simulink model "mechanization_ell_earth_noise"  (R2025b)
settings: Solver=VariableStepAuto  StartTime=0.0  StopTime=time(end)  RelTol=1e-3
values from neighbouring files (symbols this model uses):
  pqr = omega_n    [test_traj_gen_v2 1.m]    (also in test_traj_gen_v2.m)
  rpy = zeros(length(time),3)    [test_traj_gen_v2 1.m]    (also in test_traj_gen_v2.m)
  ST = 1/100    (= 0.01)    [test_traj_gen_v2 1.m]    (also in test_traj_gen_v2.m)
  vel_n = vel_n_f    [test_traj_gen_v2 1.m]    (also in test_traj_gen_v2.m)
undefined symbols (not defined in the file or in its folder): DiscIntNeverNeededParam
settings Model: Creator=Lorenzo  LastModifiedBy=roly2
settings RTWCC: GPUComputeCapability=3.5

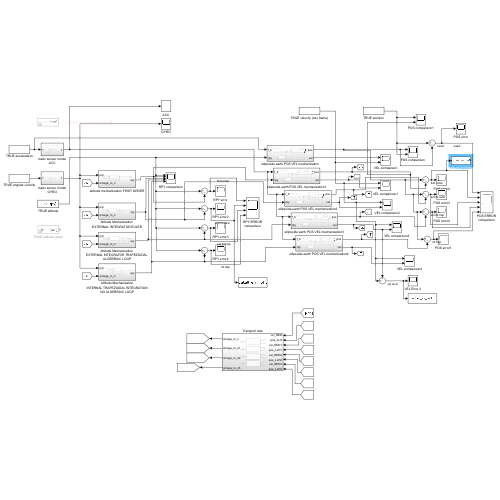
[thumbnail: Simulink's stored preview of the top-level diagram]
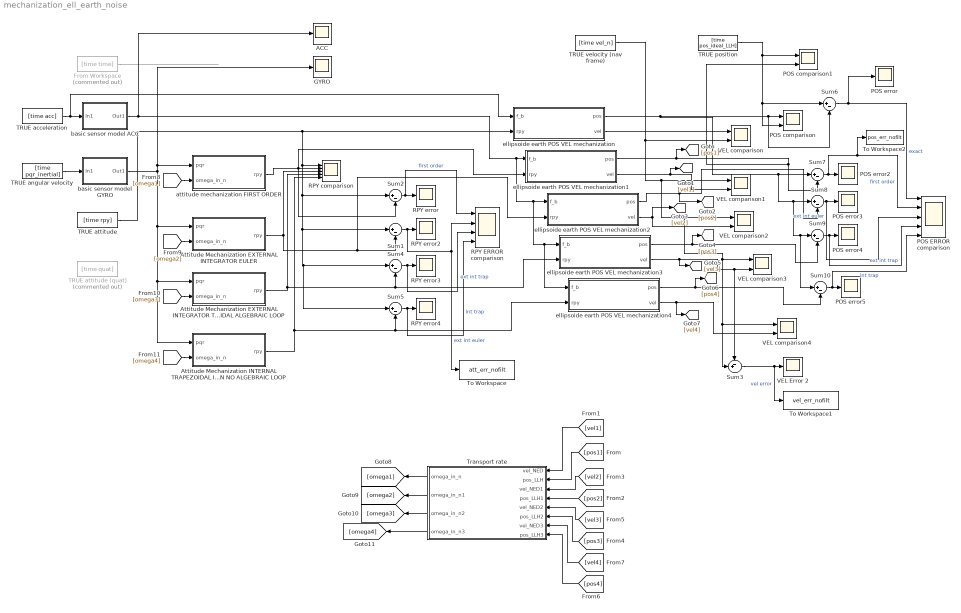
== system mechanization_ell_earth_noise ==
  ACC : Scope
      settings: ActiveDisplayYMinimum=-11.440992557737301  ActiveDisplayYMaximum=2.4820081212415044  DataLoggingVariableName=ScopeData5
  Attitude Mechanization INTERNAL TRAPEZOIDAL INTEGRATION NO ALGEBRAIC LOOP : Subsystem
  Attitude Mechanization EXTERNAL INTEGRATOR EULER : Subsystem
  Attitude Mechanization EXTERNAL INTEGRATOR TRAPEZOIDAL ALGEBRAIC LOOP : Subsystem
  From Workspace : FromWorkspace  Commented=on  VariableName=[time time]  SampleTime=ST
  GYRO : Scope
      settings: ActiveDisplayYMinimum=-0.022680320760316498  ActiveDisplayYMaximum=0.040230597398208438  DataLoggingVariableName=ScopeData12
  POS ERROR comparison : Scope  NumInputPorts=5
      settings: ActiveDisplayYMinimum=-704.98317  ActiveDisplayYMaximum=97.84622  DataLoggingVariableName=ScopeData11
  POS comparison : Scope  NumInputPorts=2
      settings: ActiveDisplayYMinimum=-2499.7198681216223  ActiveDisplayYMaximum=22499.968874235736  DataLoggingVariableName=ScopeData2
  POS comparison1 : Scope  NumInputPorts=2
      settings: ActiveDisplayYMinimum=0.69110573028876521  ActiveDisplayYMaximum=0.71972901965660918
  POS error{,2..5} (5 alike) : Scope
      POS error settings: ActiveDisplayYMinimum=-0.00026486838760320092  ActiveDisplayYMaximum=0.0023749580650473945  DataLoggingVariableName=ScopeData6
      POS error2 settings: ActiveDisplayYMinimum=-41645.7635156963  ActiveDisplayYMaximum=374810.53484694741  DataLoggingVariableName=ScopeData7
      POS error3 settings: ActiveDisplayYMinimum=-899299.95740551164  ActiveDisplayYMaximum=8.0936869298197189E+6  DataLoggingVariableName=ScopeData8
      POS error4 settings: ActiveDisplayYMinimum=-2277.2422813480371  ActiveDisplayYMaximum=2118.6339477715192  DataLoggingVariableName=ScopeData9
      POS error5 settings: ActiveDisplayYMinimum=-341009.16725  ActiveDisplayYMaximum=134356.13347  DataLoggingVariableName=ScopeData10
  RPY ERROR comparison : Scope  NumInputPorts=4
      settings: ActiveDisplayYMinimum=-1.579  ActiveDisplayYMaximum=14.13375  DataLoggingVariableName=ScopeData4
  RPY comparison : Scope  NumInputPorts=5
      settings: ActiveDisplayYMinimum=-1.2943802373057294  ActiveDisplayYMaximum=0.821675417744425
  RPY error{,2..4} (4 alike) : Scope
      RPY error settings: ActiveDisplayYMinimum=-15.337802855456003  ActiveDisplayYMaximum=8.8435208308137945
      RPY error2 settings: ActiveDisplayYMinimum=-15.811963626501008  ActiveDisplayYMaximum=3.633848239963144
      RPY error3 settings: ActiveDisplayYMinimum=-0.78598  ActiveDisplayYMaximum=7.0688  DataLoggingVariableName=ScopeData2
      RPY error4 settings: ActiveDisplayYMinimum=-16.84501  ActiveDisplayYMaximum=3.59705  DataLoggingVariableName=ScopeData3
  Sum{1..2,4..10} (9 alike) : Sum  Inputs=|+-
  Sum3 : Sum  Inputs=-+|
  TRUE acceleration : FromWorkspace  VariableName=[time acc]  SampleTime=ST
  TRUE angular velocity : FromWorkspace  VariableName=[time pqr_inertial]  SampleTime=ST
  TRUE attitude : FromWorkspace  VariableName=[time rpy]  SampleTime=ST
  TRUE attitude (quat) : FromWorkspace  Commented=on  VariableName=[time quat]
  TRUE position : FromWorkspace  VariableName=[time pos_ideal_LLH]  SampleTime=ST
  TRUE velocity (nav frame) : FromWorkspace  VariableName=[time vel_n]  SampleTime=ST
  To Workspace : ToWorkspace  VariableName=att_err_nofilt  SaveFormat=Timeseries  SampleTime=-1
  To Workspace1 : ToWorkspace  VariableName=vel_err_nofilt  SaveFormat=Timeseries  SampleTime=-1
  To Workspace2 : ToWorkspace  VariableName=pos_err_nofilt  SaveFormat=Timeseries  SampleTime=-1
  Transport rate : Subsystem
  VEL Error 2 : Scope
      settings: ActiveDisplayYMinimum=-9949.5288473837754  ActiveDisplayYMaximum=7407.62689453245  DataLoggingVariableName=ScopeData13
  VEL comparison{,1..4} (5 alike) : Scope  NumInputPorts=2
      VEL comparison settings: ActiveDisplayYMinimum=-5.5066706930115306  ActiveDisplayYMaximum=28.954763320270857  DataLoggingVariableName=ScopeData3
      VEL comparison1 settings: ActiveDisplayYMinimum=-1021.4755457862931  ActiveDisplayYMaximum=285.82124439446005  DataLoggingVariableName=ScopeData3
      VEL comparison2 settings: ActiveDisplayYMinimum=-7442.7877452030807  ActiveDisplayYMaximum=10210.805066627652  DataLoggingVariableName=ScopeData4
      VEL comparison3 settings: ActiveDisplayYMinimum=-7412.482010510731  ActiveDisplayYMaximum=9948.2828508787225  DataLoggingVariableName=ScopeData5
      VEL comparison4 settings: ActiveDisplayYMinimum=-6405.5415130223482  ActiveDisplayYMaximum=886.46101422840911  DataLoggingVariableName=ScopeData6
  attitude mechanization FIRST ORDER : Subsystem
  basic sensor model ACC : Subsystem
  basic sensor model GYRO : Subsystem
  ellipsoide earth POS VEL mechanization : Subsystem
  ellipsoide earth POS VEL mechanization1 : Subsystem
  ellipsoide earth POS VEL mechanization2 : Subsystem
  ellipsoide earth POS VEL mechanization3 : Subsystem
  ellipsoide earth POS VEL mechanization4 : Subsystem
  wires:
  From Workspace/1 -> ?
  TRUE position/1 -> POS comparison1/1, Sum6/1, POS comparison/2
  TRUE velocity (nav frame)/1 -> Sum3/2, VEL comparison4/1, VEL comparison3/1, VEL comparison2/1, VEL comparison1/1, VEL comparison/2
  Sum2/1 -> RPY ERROR comparison/1, RPY error/1  "first order"
  ellipsoide earth POS VEL mechanization/1(pos) -> Sum10/1, Sum9/1, Sum8/1, Sum7/1, Sum6/2, POS comparison/1
  ellipsoide earth POS VEL mechanization/2(vel) -> VEL comparison/1
  TRUE angular velocity/1 -> basic sensor model GYRO/1(In1)
  attitude mechanization FIRST ORDER/1(rpy) -> ellipsoide earth POS VEL mechanization1/2(rpy), Sum2/2, RPY comparison/2
  Attitude Mechanization EXTERNAL INTEGRATOR EULER/1(rpy) -> RPY comparison/3, ellipsoide earth POS VEL mechanization2/2(rpy), Sum1/2
  Sum1/1 -> To Workspace/1, RPY ERROR comparison/2, RPY error2/1  "ext int euler"
  Sum4/1 -> RPY ERROR comparison/3, RPY error3/1  "ext int trap"
  Attitude Mechanization EXTERNAL INTEGRATOR TRAPEZOIDAL ALGEBRAIC LOOP/1(rpy) -> ellipsoide earth POS VEL mechanization3/2(rpy), Sum4/2, RPY comparison/4
  Attitude Mechanization INTERNAL TRAPEZOIDAL INTEGRATION NO ALGEBRAIC LOOP/1(rpy) -> ellipsoide earth POS VEL mechanization4/2(rpy), Sum5/2, RPY comparison/5
  Sum5/1 -> RPY ERROR comparison/4, RPY error4/1  "int trap"
  TRUE attitude/1 -> Sum5/1, Sum4/1, Sum1/1, Sum2/1, RPY comparison/1, ellipsoide earth POS VEL mechanization/2(rpy)
  Sum6/1 -> POS ERROR comparison/1, POS error/1  "exact"
  Sum7/1 -> To Workspace2/1, POS ERROR comparison/2, POS error2/1  "first order"
  ellipsoide earth POS VEL mechanization1/1(pos) -> [pos1], Sum7/2, POS comparison1/2
  Sum8/1 -> POS ERROR comparison/3, POS error3/1  "ext int euler"
  ellipsoide earth POS VEL mechanization2/1(pos) -> [pos2], Sum8/2
  Sum9/1 -> POS ERROR comparison/4, POS error4/1  "ext int trap"
  ellipsoide earth POS VEL mechanization3/1(pos) -> [pos3], Sum9/2
  Sum10/1 -> POS ERROR comparison/5, POS error5/1  "int trap"
  ellipsoide earth POS VEL mechanization4/1(pos) -> [pos4], Sum10/2
  basic sensor model ACC/1(Out1) -> ACC/1, ellipsoide earth POS VEL mechanization1/1(f_b), ellipsoide earth POS VEL mechanization2/1(f_b), ellipsoide earth POS VEL mechanization4/1(f_b), ellipsoide earth POS VEL mechanization3/1(f_b)
  TRUE acceleration/1 -> ellipsoide earth POS VEL mechanization/1(f_b), basic sensor model ACC/1(In1)
  basic sensor model GYRO/1(Out1) -> GYRO/1, attitude mechanization FIRST ORDER/1(pqr), Attitude Mechanization INTERNAL TRAPEZOIDAL INTEGRATION NO ALGEBRAIC LOOP/1(pqr), Attitude Mechanization EXTERNAL INTEGRATOR TRAPEZOIDAL ALGEBRAIC LOOP/1(pqr), Attitude Mechanization EXTERNAL INTEGRATOR EULER/1(pqr)
  ellipsoide earth POS VEL mechanization1/2(vel) -> [vel1], VEL comparison1/2
  ellipsoide earth POS VEL mechanization2/2(vel) -> [vel2], VEL comparison2/2
  ellipsoide earth POS VEL mechanization3/2(vel) -> [vel3], Sum3/1, VEL comparison3/2
  ellipsoide earth POS VEL mechanization4/2(vel) -> [vel4], VEL comparison4/2
  [omega1] -> attitude mechanization FIRST ORDER/2(omega_in_n)
  [omega2] -> Attitude Mechanization EXTERNAL INTEGRATOR EULER/2(omega_in_n)
  [omega3] -> Attitude Mechanization EXTERNAL INTEGRATOR TRAPEZOIDAL ALGEBRAIC LOOP/2(omega_in_n)
  [omega4] -> Attitude Mechanization INTERNAL TRAPEZOIDAL INTEGRATION NO ALGEBRAIC LOOP/2(omega_in_n)
  [vel1] -> Transport rate/1(vel_NED)
  [pos1] -> Transport rate/2(pos_LLH)
  [vel2] -> Transport rate/3(vel_NED1)
  [pos2] -> Transport rate/4(pos_LLH1)
  [vel3] -> Transport rate/5(vel_NED2)
  [pos3] -> Transport rate/6(pos_LLH2)
  [vel4] -> Transport rate/7(vel_NED3)
  [pos4] -> Transport rate/8(pos_LLH3)
  Transport rate/1(omega_in_n) -> [omega1]
  Transport rate/2(omega_in_n1) -> [omega2]
  Transport rate/3(omega_in_n2) -> [omega3]
  Transport rate/4(omega_in_n3) -> [omega4]
  Sum3/1 -> To Workspace1/1, VEL Error 2/1  "vel error"

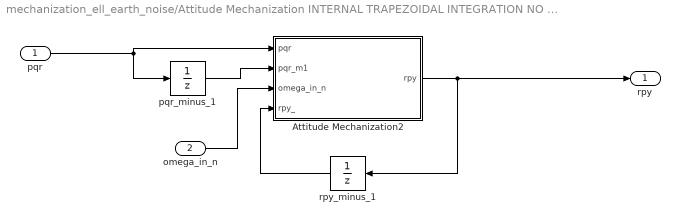
== system mechanization_ell_earth_noise/Attitude Mechanization INTERNAL TRAPEZOIDAL INTEGRATION NO ALGEBRAIC LOOP ==
  pqr : Inport
  omega_in_n : Inport  Port=2
  Attitude Mechanization2 : MATLAB Function  TreatAsAtomicUnit=on
  pqr_minus_1 : UnitDelay  InitialCondition=pqr(1,:)'  SampleTime=-1  HasFrameUpgradeWarning=on
  rpy_minus_1 : UnitDelay  InitialCondition=rpy(1,:)'  SampleTime=-1  HasFrameUpgradeWarning=on
  rpy : Outport
  wires:
  Attitude Mechanization2/1(rpy) -> rpy_minus_1/1, rpy/1
  rpy_minus_1/1 -> Attitude Mechanization2/4(rpy_)
  pqr/1 -> pqr_minus_1/1, Attitude Mechanization2/1(pqr)
  pqr_minus_1/1 -> Attitude Mechanization2/2(pqr_m1)
  omega_in_n/1 -> Attitude Mechanization2/3(omega_in_n)

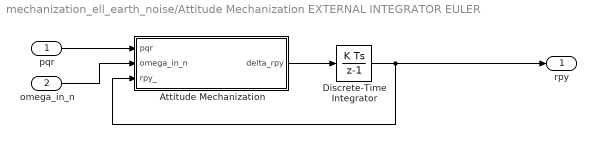
== system mechanization_ell_earth_noise/Attitude Mechanization EXTERNAL INTEGRATOR EULER ==
  pqr : Inport
  omega_in_n : Inport  Port=2
  Attitude Mechanization : MATLAB Function  TreatAsAtomicUnit=on
  Discrete-Time Integrator : DiscreteIntegrator  InitialCondition=rpy(1,:)'  SampleTime=ST  ICPrevOutput=DiscIntNeverNeededParam  ICPrevScaledInput=DiscIntNeverNeededParam
  rpy : Outport
  wires:
  Discrete-Time Integrator/1 -> rpy/1, Attitude Mechanization/3(rpy_)
  pqr/1 -> Attitude Mechanization/1(pqr)
  Attitude Mechanization/1(delta_rpy) -> Discrete-Time Integrator/1
  omega_in_n/1 -> Attitude Mechanization/2(omega_in_n)

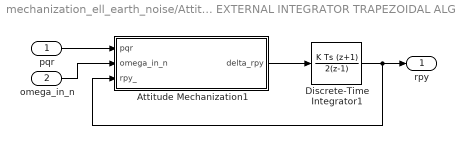
== system mechanization_ell_earth_noise/Attitude Mechanization EXTERNAL INTEGRATOR TRAPEZOIDAL ALGEBRAIC LOOP ==
  pqr : Inport
  omega_in_n : Inport  Port=2
  Attitude Mechanization1 : MATLAB Function  TreatAsAtomicUnit=on
  Discrete-Time Integrator1 : DiscreteIntegrator  IntegratorMethod=Integration: Trapezoidal  InitialCondition=rpy(1,:)'  SampleTime=ST  ICPrevOutput=DiscIntNeverNeededParam  ICPrevScaledInput=DiscIntNeverNeededParam
  rpy : Outport
  wires:
  Attitude Mechanization1/1(delta_rpy) -> Discrete-Time Integrator1/1
  pqr/1 -> Attitude Mechanization1/1(pqr)
  Discrete-Time Integrator1/1 -> Attitude Mechanization1/3(rpy_), rpy/1
  omega_in_n/1 -> Attitude Mechanization1/2(omega_in_n)

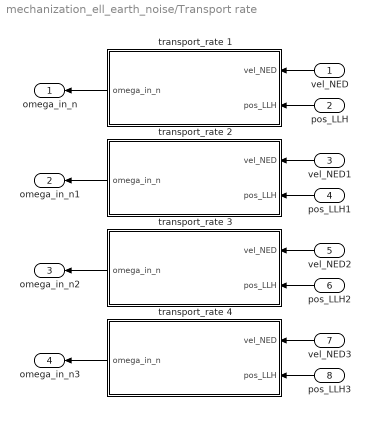
== system mechanization_ell_earth_noise/Transport rate ==
  vel_NED : Inport
  pos_LLH : Inport  Port=2
  vel_NED1 : Inport  Port=3
  pos_LLH1 : Inport  Port=4
  vel_NED2 : Inport  Port=5
  pos_LLH2 : Inport  Port=6
  vel_NED3 : Inport  Port=7
  pos_LLH3 : Inport  Port=8
  transport_rate 1 : MATLAB Function  TreatAsAtomicUnit=on
  transport_rate 2 : MATLAB Function  TreatAsAtomicUnit=on
  transport_rate 3 : MATLAB Function  TreatAsAtomicUnit=on
  transport_rate 4 : MATLAB Function  TreatAsAtomicUnit=on
  omega_in_n : Outport
  omega_in_n1 : Outport  Port=2
  omega_in_n2 : Outport  Port=3
  omega_in_n3 : Outport  Port=4
  wires:
  pos_LLH2/1 -> transport_rate 3/2(pos_LLH)
  transport_rate 4/1(omega_in_n) -> omega_in_n3/1
  pos_LLH/1 -> transport_rate 1/2(pos_LLH)
  vel_NED/1 -> transport_rate 1/1(vel_NED)
  pos_LLH3/1 -> transport_rate 4/2(pos_LLH)
  vel_NED3/1 -> transport_rate 4/1(vel_NED)
  transport_rate 3/1(omega_in_n) -> omega_in_n2/1
  pos_LLH1/1 -> transport_rate 2/2(pos_LLH)
  transport_rate 2/1(omega_in_n) -> omega_in_n1/1
  transport_rate 1/1(omega_in_n) -> omega_in_n/1
  vel_NED1/1 -> transport_rate 2/1(vel_NED)
  vel_NED2/1 -> transport_rate 3/1(vel_NED)

== system mechanization_ell_earth_noise/attitude mechanization FIRST ORDER ==
  pqr : Inport
  omega_in_n : Inport  Port=2
  Attitude Mechanization : MATLAB Function  TreatAsAtomicUnit=on
  rpy_mem : UnitDelay  InitialCondition=rpy(1,:)'  SampleTime=-1  HasFrameUpgradeWarning=on
  rpy : Outport
  wires:
  pqr/1 -> Attitude Mechanization/1(pqr)
  rpy_mem/1 -> Attitude Mechanization/3(rpy_)
  Attitude Mechanization/1(rpy) -> rpy_mem/1, rpy/1
  omega_in_n/1 -> Attitude Mechanization/2(omega_in_n)

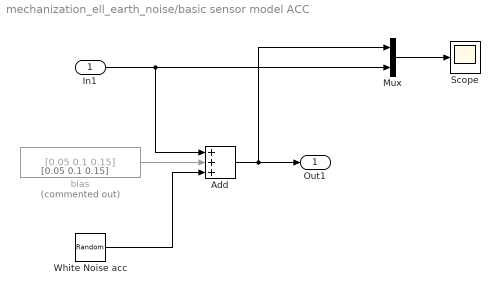
== system mechanization_ell_earth_noise/basic sensor model ACC ==
  note: [0.05 0.1 0.15]
  In1 : Inport
  Add : Sum  Inputs=+++
  Mux : Mux  Inputs=2
  Scope : Scope
      settings: ActiveDisplayYMinimum=-0.7520653966044506  ActiveDisplayYMaximum=0.75172983316287767
  White Noise acc : RandomNumber  DisableCoverage=on  Mean=[0 0 0 ]  Variance=[0.05 0.05 0.05].^2  Seed=[1 2 3]  SampleTime=ST
  bias : Constant  Commented=on  Value=[0.05 0.1 0.15]
  Out1 : Outport
  wires:
  In1/1 -> Mux/2, Add/1
  White Noise acc/1 -> Add/3
  bias/1 -> Add/2
  Mux/1 -> Scope/1
  Add/1 -> Mux/1, Out1/1

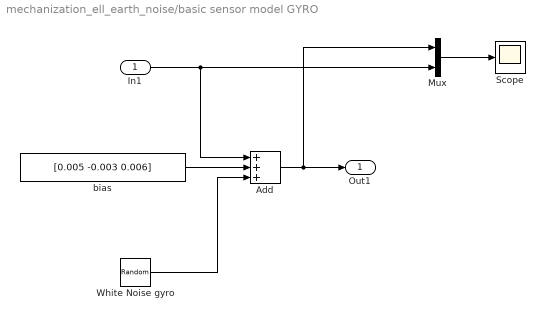
== system mechanization_ell_earth_noise/basic sensor model GYRO ==
  In1 : Inport
  Add : Sum  Inputs=+++
  Mux : Mux  Inputs=2
  Scope : Scope
      settings: ActiveDisplayYMinimum=-0.018561300716746276  ActiveDisplayYMaximum=0.027069948726320941  DataLoggingVariableName=ScopeData2
  White Noise gyro : RandomNumber  DisableCoverage=on  Mean=[0 0 0]  Variance=[0.003 0.003 0.003].^2  Seed=[4 5 6]  SampleTime=ST
  bias : Constant  Value=[0.005 -0.003 0.006]
  Out1 : Outport
  wires:
  White Noise gyro/1 -> Add/3
  bias/1 -> Add/2
  Mux/1 -> Scope/1
  In1/1 -> Mux/2, Add/1
  Add/1 -> Mux/1, Out1/1

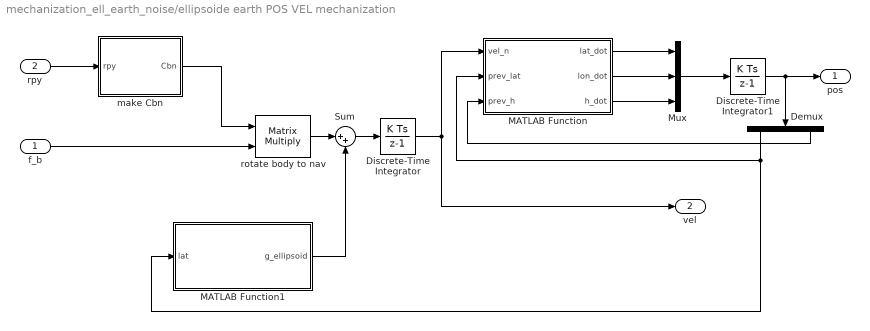
== system mechanization_ell_earth_noise/ellipsoide earth POS VEL mechanization ==
  f_b : Inport
  rpy : Inport  Port=2
  Demux : Demux  Outputs=3
  Discrete-Time Integrator : DiscreteIntegrator  InitialCondition=vel_n(1,:)  SampleTime=-1  ICPrevOutput=DiscIntNeverNeededParam  ICPrevScaledInput=DiscIntNeverNeededParam
  Discrete-Time Integrator1 : DiscreteIntegrator  InitialCondition=[40.8522 * pi/180 ; 14.2681 * pi/180 ; 20000]  SampleTime=-1  ICPrevOutput=DiscIntNeverNeededParam  ICPrevScaledInput=DiscIntNeverNeededParam
  MATLAB Function : MATLAB Function  TreatAsAtomicUnit=on
  MATLAB Function1 : MATLAB Function  TreatAsAtomicUnit=on
  Mux : Mux  Inputs=3
  Sum : Sum  Inputs=|++
  make Cbn : MATLAB Function  TreatAsAtomicUnit=on
  rotate body to nav : Product  Multiplication=Matrix(*)
  pos : Outport
  vel : Outport  Port=2
  wires:
  rotate body to nav/1 -> Sum/1
  MATLAB Function1/1(g_ellipsoid) -> Sum/2
  Discrete-Time Integrator/1 -> MATLAB Function/1(vel_n), vel/1
  make Cbn/1(Cbn) -> rotate body to nav/1
  Sum/1 -> Discrete-Time Integrator/1
  f_b/1 -> rotate body to nav/2
  rpy/1 -> make Cbn/1(rpy)
  MATLAB Function/3(h_dot) -> Mux/3
  MATLAB Function/2(lon_dot) -> Mux/2
  MATLAB Function/1(lat_dot) -> Mux/1
  Mux/1 -> Discrete-Time Integrator1/1
  Discrete-Time Integrator1/1 -> pos/1, Demux/1
  Demux/1 -> MATLAB Function1/1(lat), MATLAB Function/2(prev_lat)
  Demux/3 -> MATLAB Function/3(prev_h)

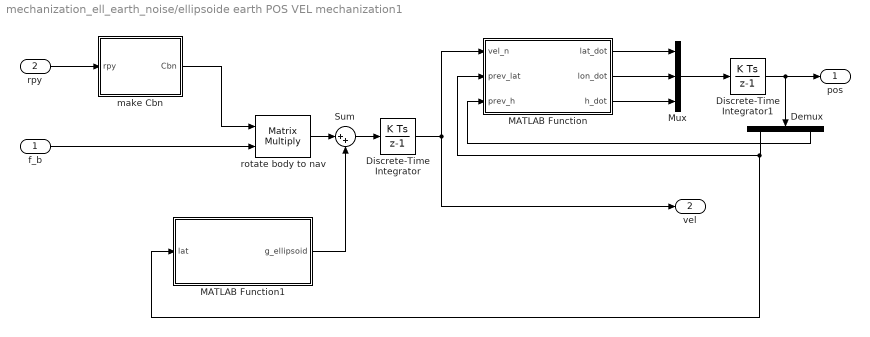
== system mechanization_ell_earth_noise/ellipsoide earth POS VEL mechanization1 ==
  f_b : Inport
  rpy : Inport  Port=2
  Demux : Demux  Outputs=3
  Discrete-Time Integrator : DiscreteIntegrator  InitialCondition=vel_n(1,:)  SampleTime=-1  ICPrevOutput=DiscIntNeverNeededParam  ICPrevScaledInput=DiscIntNeverNeededParam
  Discrete-Time Integrator1 : DiscreteIntegrator  InitialCondition=[40.8522 * pi/180 ; 14.2681 * pi/180 ; 20000]  SampleTime=-1  ICPrevOutput=DiscIntNeverNeededParam  ICPrevScaledInput=DiscIntNeverNeededParam
  MATLAB Function : MATLAB Function  TreatAsAtomicUnit=on
  MATLAB Function1 : MATLAB Function  TreatAsAtomicUnit=on
  Mux : Mux  Inputs=3
  Sum : Sum  Inputs=|++
  make Cbn : MATLAB Function  TreatAsAtomicUnit=on
  rotate body to nav : Product  Multiplication=Matrix(*)
  pos : Outport
  vel : Outport  Port=2
  wires:
  rotate body to nav/1 -> Sum/1
  Discrete-Time Integrator/1 -> MATLAB Function/1(vel_n), vel/1
  make Cbn/1(Cbn) -> rotate body to nav/1
  Sum/1 -> Discrete-Time Integrator/1
  f_b/1 -> rotate body to nav/2
  rpy/1 -> make Cbn/1(rpy)
  MATLAB Function/3(h_dot) -> Mux/3
  MATLAB Function/2(lon_dot) -> Mux/2
  MATLAB Function/1(lat_dot) -> Mux/1
  Mux/1 -> Discrete-Time Integrator1/1
  Discrete-Time Integrator1/1 -> pos/1, Demux/1
  Demux/3 -> MATLAB Function/3(prev_h)
  Demux/1 -> MATLAB Function1/1(lat), MATLAB Function/2(prev_lat)
  MATLAB Function1/1(g_ellipsoid) -> Sum/2

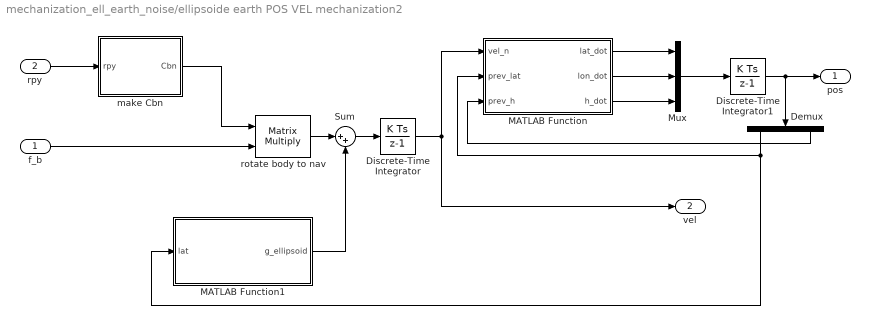
== system mechanization_ell_earth_noise/ellipsoide earth POS VEL mechanization2 ==
  f_b : Inport
  rpy : Inport  Port=2
  Demux : Demux  Outputs=3
  Discrete-Time Integrator : DiscreteIntegrator  InitialCondition=vel_n(1,:)  SampleTime=-1  ICPrevOutput=DiscIntNeverNeededParam  ICPrevScaledInput=DiscIntNeverNeededParam
  Discrete-Time Integrator1 : DiscreteIntegrator  InitialCondition=[40.8522 * pi/180 ; 14.2681 * pi/180 ; 20000]  SampleTime=-1  ICPrevOutput=DiscIntNeverNeededParam  ICPrevScaledInput=DiscIntNeverNeededParam
  MATLAB Function : MATLAB Function  TreatAsAtomicUnit=on
  MATLAB Function1 : MATLAB Function  TreatAsAtomicUnit=on
  Mux : Mux  Inputs=3
  Sum : Sum  Inputs=|++
  make Cbn : MATLAB Function  TreatAsAtomicUnit=on
  rotate body to nav : Product  Multiplication=Matrix(*)
  pos : Outport
  vel : Outport  Port=2
  wires:
  rotate body to nav/1 -> Sum/1
  Discrete-Time Integrator/1 -> MATLAB Function/1(vel_n), vel/1
  make Cbn/1(Cbn) -> rotate body to nav/1
  Sum/1 -> Discrete-Time Integrator/1
  f_b/1 -> rotate body to nav/2
  rpy/1 -> make Cbn/1(rpy)
  MATLAB Function/3(h_dot) -> Mux/3
  MATLAB Function/2(lon_dot) -> Mux/2
  MATLAB Function/1(lat_dot) -> Mux/1
  Mux/1 -> Discrete-Time Integrator1/1
  Discrete-Time Integrator1/1 -> pos/1, Demux/1
  Demux/3 -> MATLAB Function/3(prev_h)
  Demux/1 -> MATLAB Function1/1(lat), MATLAB Function/2(prev_lat)
  MATLAB Function1/1(g_ellipsoid) -> Sum/2

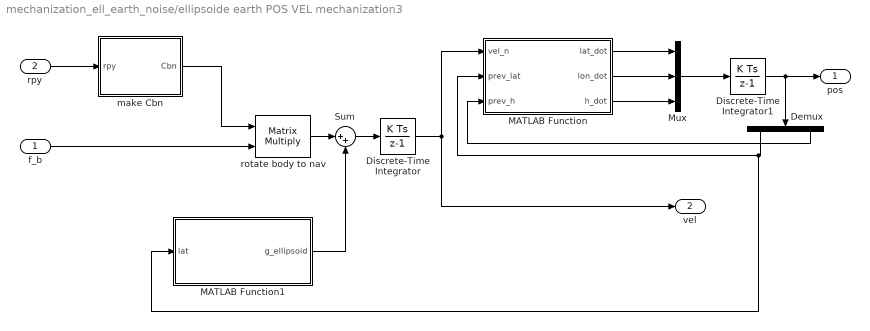
== system mechanization_ell_earth_noise/ellipsoide earth POS VEL mechanization3 ==
  f_b : Inport
  rpy : Inport  Port=2
  Demux : Demux  Outputs=3
  Discrete-Time Integrator : DiscreteIntegrator  InitialCondition=vel_n(1,:)  SampleTime=-1  ICPrevOutput=DiscIntNeverNeededParam  ICPrevScaledInput=DiscIntNeverNeededParam
  Discrete-Time Integrator1 : DiscreteIntegrator  InitialCondition=[40.8522 * pi/180 ; 14.2681 * pi/180 ; 20000]  SampleTime=-1  ICPrevOutput=DiscIntNeverNeededParam  ICPrevScaledInput=DiscIntNeverNeededParam
  MATLAB Function : MATLAB Function  TreatAsAtomicUnit=on
  MATLAB Function1 : MATLAB Function  TreatAsAtomicUnit=on
  Mux : Mux  Inputs=3
  Sum : Sum  Inputs=|++
  make Cbn : MATLAB Function  TreatAsAtomicUnit=on
  rotate body to nav : Product  Multiplication=Matrix(*)
  pos : Outport
  vel : Outport  Port=2
  wires:
  rotate body to nav/1 -> Sum/1
  Discrete-Time Integrator/1 -> MATLAB Function/1(vel_n), vel/1
  make Cbn/1(Cbn) -> rotate body to nav/1
  Sum/1 -> Discrete-Time Integrator/1
  f_b/1 -> rotate body to nav/2
  rpy/1 -> make Cbn/1(rpy)
  MATLAB Function/3(h_dot) -> Mux/3
  MATLAB Function/2(lon_dot) -> Mux/2
  MATLAB Function/1(lat_dot) -> Mux/1
  Mux/1 -> Discrete-Time Integrator1/1
  Discrete-Time Integrator1/1 -> pos/1, Demux/1
  Demux/3 -> MATLAB Function/3(prev_h)
  Demux/1 -> MATLAB Function1/1(lat), MATLAB Function/2(prev_lat)
  MATLAB Function1/1(g_ellipsoid) -> Sum/2

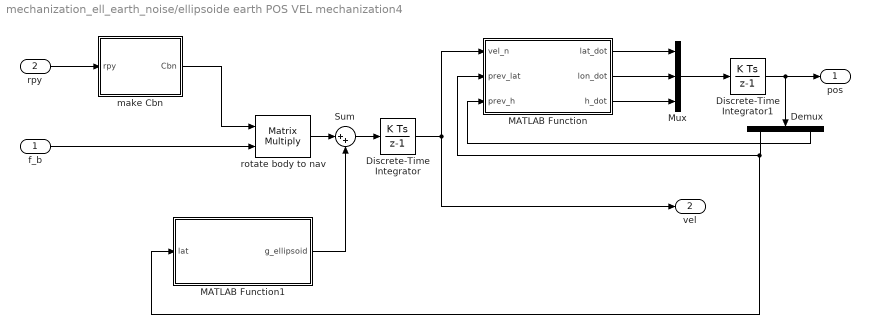
== system mechanization_ell_earth_noise/ellipsoide earth POS VEL mechanization4 ==
  f_b : Inport
  rpy : Inport  Port=2
  Demux : Demux  Outputs=3
  Discrete-Time Integrator : DiscreteIntegrator  InitialCondition=vel_n(1,:)  SampleTime=-1  ICPrevOutput=DiscIntNeverNeededParam  ICPrevScaledInput=DiscIntNeverNeededParam
  Discrete-Time Integrator1 : DiscreteIntegrator  InitialCondition=[40.8522 * pi/180 ; 14.2681 * pi/180 ; 20000]  SampleTime=-1  ICPrevOutput=DiscIntNeverNeededParam  ICPrevScaledInput=DiscIntNeverNeededParam
  MATLAB Function : MATLAB Function  TreatAsAtomicUnit=on
  MATLAB Function1 : MATLAB Function  TreatAsAtomicUnit=on
  Mux : Mux  Inputs=3
  Sum : Sum  Inputs=|++
  make Cbn : MATLAB Function  TreatAsAtomicUnit=on
  rotate body to nav : Product  Multiplication=Matrix(*)
  pos : Outport
  vel : Outport  Port=2
  wires:
  rotate body to nav/1 -> Sum/1
  Discrete-Time Integrator/1 -> MATLAB Function/1(vel_n), vel/1
  make Cbn/1(Cbn) -> rotate body to nav/1
  Sum/1 -> Discrete-Time Integrator/1
  f_b/1 -> rotate body to nav/2
  rpy/1 -> make Cbn/1(rpy)
  MATLAB Function/3(h_dot) -> Mux/3
  MATLAB Function/2(lon_dot) -> Mux/2
  MATLAB Function/1(lat_dot) -> Mux/1
  Mux/1 -> Discrete-Time Integrator1/1
  Discrete-Time Integrator1/1 -> pos/1, Demux/1
  Demux/3 -> MATLAB Function/3(prev_h)
  Demux/1 -> MATLAB Function1/1(lat), MATLAB Function/2(prev_lat)
  MATLAB Function1/1(g_ellipsoid) -> Sum/2

== matlab function mechanization_ell_earth_noise/ellipsoide earth POS VEL mechanization/MATLAB Function ==
  data: vel_n input; lat_dot output; prev_lat input; prev_h input; lon_dot output; h_dot output
function [lat_dot, lon_dot, h_dot] = ellipsoid_mechanization(vel_n, prev_lat, prev_h)

vel_N = vel_n(1);
vel_E = vel_n(2);
vel_D = vel_n(3);

% Constants WGS-84

re = 6378137;
eps = 0.0818191908426;
eps2 = eps^2;

phi = prev_lat;
h = prev_h;

sin2phi = sin(phi)^2;
den = 1 - eps2 * sin2phi ; 

R_N = re / (sqrt(den));
R_M = R_N * (1 - eps2)/(den);

lat_dot = vel_N / (R_M + h);
lon_dot = vel_E / (R_N + h) / cos(phi) ;
h_dot = - vel_D;

end

== matlab function mechanization_ell_earth_noise/ellipsoide earth POS VEL mechanization1/make Cbn ==
  data: rpy input; Cbn output
function Cbn = make_Cbn(rpy)
%compute Cbn
Cz=[cos(rpy(3))     sin(rpy(3))     0; ...
    -sin(rpy(3))    cos(rpy(3))     0; ...
    0               0               1];

Cy=[cos(rpy(2))     0               -sin(rpy(2)); ...
    0               1               0; ...
    sin(rpy(2))     0               cos(rpy(2))];

Cx=[1               0               0;...
    0               cos(rpy(1))     sin(rpy(1)); ...
    0               -sin(rpy(1))    cos(rpy(1))];

Cbn = (Cx*Cy*Cz)';

== matlab function mechanization_ell_earth_noise/ellipsoide earth POS VEL mechanization3/make Cbn ==
  data: rpy input; Cbn output
function Cbn = make_Cbn(rpy)
%compute Cbn
Cz=[cos(rpy(3))     sin(rpy(3))     0; ...
    -sin(rpy(3))    cos(rpy(3))     0; ...
    0               0               1];

Cy=[cos(rpy(2))     0               -sin(rpy(2)); ...
    0               1               0; ...
    sin(rpy(2))     0               cos(rpy(2))];

Cx=[1               0               0;...
    0               cos(rpy(1))     sin(rpy(1)); ...
    0               -sin(rpy(1))    cos(rpy(1))];

Cbn = (Cx*Cy*Cz)';

== matlab function mechanization_ell_earth_noise/ellipsoide earth POS VEL mechanization1/MATLAB Function ==
  data: vel_n input; lat_dot output; prev_lat input; prev_h input; lon_dot output; h_dot output
function [lat_dot, lon_dot, h_dot] = ellipsoid_mechanization(vel_n, prev_lat, prev_h)

vel_N = vel_n(1);
vel_E = vel_n(2);
vel_D = vel_n(3);

% Constants WGS-84

re = 6378137;
eps = 0.0818191908426;
eps2 = eps^2;

phi = prev_lat;
h = prev_h;

sin2phi = sin(phi)^2;
den = 1 - eps2 * sin2phi ; 

R_N = re / (sqrt(den));
R_M = R_N * (1 - eps2)/(den);

lat_dot = vel_N / (R_M + h);
lon_dot = vel_E / (R_N + h) / cos(phi) ;
h_dot = - vel_D;

end

== matlab function mechanization_ell_earth_noise/ellipsoide earth POS VEL mechanization4/MATLAB Function ==
  data: vel_n input; lat_dot output; prev_lat input; prev_h input; lon_dot output; h_dot output
function [lat_dot, lon_dot, h_dot] = ellipsoid_mechanization(vel_n, prev_lat, prev_h)

vel_N = vel_n(1);
vel_E = vel_n(2);
vel_D = vel_n(3);

% Constants WGS-84

re = 6378137;
eps = 0.0818191908426;
eps2 = eps^2;

phi = prev_lat;
h = prev_h;

sin2phi = sin(phi)^2;
den = 1 - eps2 * sin2phi ; 

R_N = re / (sqrt(den));
R_M = R_N * (1 - eps2)/(den);

lat_dot = vel_N / (R_M + h);
lon_dot = vel_E / (R_N + h) / cos(phi) ;
h_dot = - vel_D;

end

== matlab function mechanization_ell_earth_noise/ellipsoide earth POS VEL mechanization4/make Cbn ==
  data: rpy input; Cbn output
function Cbn = make_Cbn(rpy)
%compute Cbn
Cz=[cos(rpy(3))     sin(rpy(3))     0; ...
    -sin(rpy(3))    cos(rpy(3))     0; ...
    0               0               1];

Cy=[cos(rpy(2))     0               -sin(rpy(2)); ...
    0               1               0; ...
    sin(rpy(2))     0               cos(rpy(2))];

Cx=[1               0               0;...
    0               cos(rpy(1))     sin(rpy(1)); ...
    0               -sin(rpy(1))    cos(rpy(1))];

Cbn = (Cx*Cy*Cz)';

== matlab function mechanization_ell_earth_noise/Transport rate/transport_rate 1 ==
  data: vel_NED input; omega_in_n output; pos_LLH input
function omega_in_n = transport_rate(vel_NED, pos_LLH)

v_N = vel_NED(1);
v_E = vel_NED(2);

phi = pos_LLH(1);
h = pos_LLH(3);

omega_E = 7.292115e-5; % Velocità di rotazione terrestre [rad/s]

re = 6378137;
eps = 0.0818191908426;
eps2 = eps^2;

sin2phi = sin(phi)^2;
den = 1 - eps2 * sin2phi;
R_N = re / (sqrt(den));
R_M = R_N * (1 - eps2) / den;

omega_ie_n = [omega_E * cos(phi) ; 0; -omega_E * sin(phi)];

omega_en_n = [  v_E / (R_N + h);
                -v_N / (R_M + h);
                -v_E * tan(phi) / (R_N + h)];

omega_in_n = omega_ie_n + omega_en_n;

end

== matlab function mechanization_ell_earth_noise/Transport rate/transport_rate 2 ==
  data: vel_NED input; omega_in_n output; pos_LLH input
function omega_in_n = transport_rate(vel_NED, pos_LLH)

v_N = vel_NED(1);
v_E = vel_NED(2);

phi = pos_LLH(1);
h = pos_LLH(3);

omega_E = 7.292115e-5; % Velocità di rotazione terrestre [rad/s]

re = 6378137;
eps = 0.0818191908426;
eps2 = eps^2;

sin2phi = sin(phi)^2;
den = 1 - eps2 * sin2phi;
R_N = re / (sqrt(den));
R_M = R_N * (1 - eps2) / den;

omega_ie_n = [omega_E * cos(phi) ; 0; -omega_E * sin(phi)];

omega_en_n = [  v_E / (R_N + h);
                -v_N / (R_M + h);
                -v_E * tan(phi) / (R_N + h)];

omega_in_n = omega_ie_n + omega_en_n;

end

== matlab function mechanization_ell_earth_noise/Transport rate/transport_rate 3 ==
  data: vel_NED input; omega_in_n output; pos_LLH input
function omega_in_n = transport_rate(vel_NED, pos_LLH)

v_N = vel_NED(1);
v_E = vel_NED(2);

phi = pos_LLH(1);
h = pos_LLH(3);

omega_E = 7.292115e-5; % Velocità di rotazione terrestre [rad/s]

re = 6378137;
eps = 0.0818191908426;
eps2 = eps^2;

sin2phi = sin(phi)^2;
den = 1 - eps2 * sin2phi;
R_N = re / (sqrt(den));
R_M = R_N * (1 - eps2) / den;

omega_ie_n = [omega_E * cos(phi) ; 0; -omega_E * sin(phi)];

omega_en_n = [  v_E / (R_N + h);
                -v_N / (R_M + h);
                -v_E * tan(phi) / (R_N + h)];

omega_in_n = omega_ie_n + omega_en_n;

end

== matlab function mechanization_ell_earth_noise/Transport rate/transport_rate 4 ==
  data: vel_NED input; omega_in_n output; pos_LLH input
function omega_in_n = transport_rate(vel_NED, pos_LLH)

v_N = vel_NED(1);
v_E = vel_NED(2);

phi = pos_LLH(1);
h = pos_LLH(3);

omega_E = 7.292115e-5; % Velocità di rotazione terrestre [rad/s]

re = 6378137;
eps = 0.0818191908426;
eps2 = eps^2;

sin2phi = sin(phi)^2;
den = 1 - eps2 * sin2phi;
R_N = re / (sqrt(den));
R_M = R_N * (1 - eps2) / den;

omega_ie_n = [omega_E * cos(phi) ; 0; -omega_E * sin(phi)];

omega_en_n = [  v_E / (R_N + h);
                -v_N / (R_M + h);
                -v_E * tan(phi) / (R_N + h)];

omega_in_n = omega_ie_n + omega_en_n;

end

== matlab function mechanization_ell_earth_noise/ellipsoide earth POS VEL mechanization/MATLAB Function1 ==
  data: lat input; g_ellipsoid output
function g_ellipsoid = gravity_compansation(lat)

g_wgs0 = 9.7803267714;
g_wgs1 = 0.00193185138639;

eps = 0.0818191908426;
eps2 = eps^2;

sin2phi = sin(lat)^2;
g = g_wgs0 * (1 + g_wgs1 * sin2phi) / sqrt(1 - eps2 * sin2phi);
g_ellipsoid = [0; 0; g];

== matlab function mechanization_ell_earth_noise/ellipsoide earth POS VEL mechanization1/MATLAB Function1 ==
  data: lat input; g_ellipsoid output
function g_ellipsoid = gravity_compansation(lat)

g_wgs0 = 9.7803267714;
g_wgs1 = 0.00193185138639;

eps = 0.0818191908426;
eps2 = eps^2;

sin2phi = sin(lat)^2;
g = g_wgs0 * (1 + g_wgs1 * sin2phi) / sqrt(1 - eps2 * sin2phi);
g_ellipsoid = [0; 0; g];

== matlab function mechanization_ell_earth_noise/ellipsoide earth POS VEL mechanization2/MATLAB Function1 ==
  data: lat input; g_ellipsoid output
function g_ellipsoid = gravity_compansation(lat)

g_wgs0 = 9.7803267714;
g_wgs1 = 0.00193185138639;

eps = 0.0818191908426;
eps2 = eps^2;

sin2phi = sin(lat)^2;
g = g_wgs0 * (1 + g_wgs1 * sin2phi) / sqrt(1 - eps2 * sin2phi);
g_ellipsoid = [0; 0; g];

== matlab function mechanization_ell_earth_noise/ellipsoide earth POS VEL mechanization3/MATLAB Function1 ==
  data: lat input; g_ellipsoid output
function g_ellipsoid = gravity_compansation(lat)

g_wgs0 = 9.7803267714;
g_wgs1 = 0.00193185138639;

eps = 0.0818191908426;
eps2 = eps^2;

sin2phi = sin(lat)^2;
g = g_wgs0 * (1 + g_wgs1 * sin2phi) / sqrt(1 - eps2 * sin2phi);
g_ellipsoid = [0; 0; g];

== matlab function mechanization_ell_earth_noise/ellipsoide earth POS VEL mechanization4/MATLAB Function1 ==
  data: lat input; g_ellipsoid output
function g_ellipsoid = gravity_compansation(lat)

g_wgs0 = 9.7803267714;
g_wgs1 = 0.00193185138639;

eps = 0.0818191908426;
eps2 = eps^2;

sin2phi = sin(lat)^2;
g = g_wgs0 * (1 + g_wgs1 * sin2phi) / sqrt(1 - eps2 * sin2phi);
g_ellipsoid = [0; 0; g];

== matlab function mechanization_ell_earth_noise/attitude mechanization FIRST ORDER/Attitude Mechanization ==
  data: pqr input; omega_in_n input; rpy output; rpy_ input; ST parameter size=1
function rpy = attitude_mech(pqr, omega_in_n, rpy_,ST)
%input:angular velocity at current timestep, latest estimation of attitude
%output> rpy and Cbn

phi = rpy_(1); 
theta = rpy_(2); 
psi = rpy_(3);

% Calculate C_n_b

cph = cos(phi);   sph = sin(phi);
cth = cos(theta); sth = sin(theta);
cps = cos(psi);   sps = sin(psi);

C_b_n = [cth*cps,  sph*sth*cps - cph*sps,  cph*sth*cps + sph*sps;
         cth*sps,  sph*sth*sps + cph*cps,  cph*sth*sps - sph*cps;
         -sth,     sph*cth,                cph*cth];
C_n_b = C_b_n';

% Transport rate correction

pqr_corrected = pqr - C_n_b * omega_in_n;

%create Jacobian that transforms angular rates into rates of Euler
%angles
J = [1, sin(phi)*tan(theta), cos(phi)*tan(theta);
     0, cos(phi),            -sin(phi);
     0, sin(phi)/cos(theta), cos(phi)/cos(theta)];

%integrate
delta_rpy = J*pqr_corrected*ST;

rpy=rpy_ + delta_rpy;

== matlab function mechanization_ell_earth_noise/ellipsoide earth POS VEL mechanization2/MATLAB Function ==
  data: vel_n input; lat_dot output; prev_lat input; prev_h input; lon_dot output; h_dot output
function [lat_dot, lon_dot, h_dot] = ellipsoid_mechanization(vel_n, prev_lat, prev_h)

vel_N = vel_n(1);
vel_E = vel_n(2);
vel_D = vel_n(3);

% Constants WGS-84

re = 6378137;
eps = 0.0818191908426;
eps2 = eps^2;

phi = prev_lat;
h = prev_h;

sin2phi = sin(phi)^2;
den = 1 - eps2 * sin2phi ; 

R_N = re / (sqrt(den));
R_M = R_N * (1 - eps2)/(den);

lat_dot = vel_N / (R_M + h);
lon_dot = vel_E / (R_N + h) / cos(phi) ;
h_dot = - vel_D;

end

== matlab function mechanization_ell_earth_noise/Attitude Mechanization EXTERNAL INTEGRATOR EULER/Attitude Mechanization ==
  data: pqr input; omega_in_n input; delta_rpy output; rpy_ input; ST parameter size=1
function delta_rpy = attitude_mech(pqr, omega_in_n, rpy_,ST)
%input:angular velocity at current timestep, latest estimation of attitude
%output> rpy and Cbn

phi = rpy_(1); 
theta = rpy_(2);
psi = rpy_(3);

% Calculate C_n_b

cph = cos(phi);   sph = sin(phi);
cth = cos(theta); sth = sin(theta);
cps = cos(psi);   sps = sin(psi);

C_b_n = [cth*cps,  sph*sth*cps - cph*sps,  cph*sth*cps + sph*sps;
         cth*sps,  sph*sth*sps + cph*cps,  cph*sth*sps - sph*cps;
         -sth,     sph*cth,                cph*cth];
C_n_b = C_b_n';

% Transport rate correction

pqr_corrected = pqr - C_n_b * omega_in_n;
%create Jacobian that transforms angular rates into rates of Euler
%angles
J = [1, sin(phi)*tan(theta), cos(phi)*tan(theta);
     0, cos(phi),            -sin(phi);
     0, sin(phi)/cos(theta), cos(phi)/cos(theta)];

%integrate
delta_rpy = J*pqr_corrected;

== matlab function mechanization_ell_earth_noise/Attitude Mechanization EXTERNAL INTEGRATOR TRAPEZOIDAL ALGEBRAIC LOOP/Attitude Mechanization1 ==
  data: pqr input; omega_in_n input; delta_rpy output; rpy_ input; ST parameter size=1
function delta_rpy = attitude_mech(pqr,omega_in_n, rpy_,ST)
%input:angular velocity at current timestep, latest estimation of attitude
%output> rpy and Cbn

phi = rpy_(1); 
theta = rpy_(2); 
psi = rpy_(3);

% Calculate C_n_b

cph = cos(phi);   sph = sin(phi);
cth = cos(theta); sth = sin(theta);
cps = cos(psi);   sps = sin(psi);

C_b_n = [cth*cps,  sph*sth*cps - cph*sps,  cph*sth*cps + sph*sps;
         cth*sps,  sph*sth*sps + cph*cps,  cph*sth*sps - sph*cps;
         -sth,     sph*cth,                cph*cth];
C_n_b = C_b_n';

% Transport rate correction

pqr_corrected = pqr - C_n_b * omega_in_n;
%create Jacobian that transforms angular rates into rates of Euler
%angles
J = [1, sin(phi)*tan(theta), cos(phi)*tan(theta);
     0, cos(phi),            -sin(phi);
     0, sin(phi)/cos(theta), cos(phi)/cos(theta)];

%integrate
delta_rpy = J*pqr_corrected;

== matlab function mechanization_ell_earth_noise/ellipsoide earth POS VEL mechanization/make Cbn ==
  data: rpy input; Cbn output
function Cbn = make_Cbn(rpy)
%compute Cbn
Cz=[cos(rpy(3))     sin(rpy(3))     0; ...
    -sin(rpy(3))    cos(rpy(3))     0; ...
    0               0               1];

Cy=[cos(rpy(2))     0               -sin(rpy(2)); ...
    0               1               0; ...
    sin(rpy(2))     0               cos(rpy(2))];

Cx=[1               0               0;...
    0               cos(rpy(1))     sin(rpy(1)); ...
    0               -sin(rpy(1))    cos(rpy(1))];

Cbn = (Cx*Cy*Cz)';

== matlab function mechanization_ell_earth_noise/Attitude Mechanization INTERNAL TRAPEZOIDAL INTEGRATION NO ALGEBRAIC LOOP/Attitude Mechanization2 ==
  data: pqr input; pqr_m1 input; omega_in_n input; rpy output; rpy_ input; ST parameter size=1
function rpy = attitude_mech(pqr, pqr_m1, omega_in_n, rpy_,ST)
%input:angular velocity at current timestep, latest estimation of attitude
%output> rpy and Cbn

phi = rpy_(1); 
theta = rpy_(2);
psi = rpy_(3);

% Calculate C_n_b

cph = cos(phi);   sph = sin(phi);
cth = cos(theta); sth = sin(theta);
cps = cos(psi);   sps = sin(psi);

C_b_n = [cth*cps,  sph*sth*cps - cph*sps,  cph*sth*cps + sph*sps;
         cth*sps,  sph*sth*sps + cph*cps,  cph*sth*sps - sph*cps;
         -sth,     sph*cth,                cph*cth];
C_n_b = C_b_n';

% Transport rate correction

pqr_corrected = pqr - C_n_b * omega_in_n;
pqr_m1_corrected = pqr_m1 - C_n_b * omega_in_n;

%create Jacobian that transforms angular rates into rates of Euler
%angles
J = [1, sin(phi)*tan(theta), cos(phi)*tan(theta);
     0, cos(phi),            -sin(phi);
     0, sin(phi)/cos(theta), cos(phi)/cos(theta)];
delta_rpy_m1 = J*pqr_m1_corrected*ST;

%integrate one step forward
rpy=rpy_ + delta_rpy_m1;

%get new euler angles and compute angle derivatives one step forward 
phi = rpy(1); 
theta = rpy(2); 
%create Jacobian that transforms angular rates into rates of Euler
%angles
J = [1, sin(phi)*tan(theta), cos(phi)*tan(theta);
     0, cos(phi),            -sin(phi);
     0, sin(phi)/cos(theta), cos(phi)/cos(theta)];
delta_rpy=J*pqr_corrected*ST;

%perform trapezoidal integration
rpy=rpy_ + (delta_rpy + delta_rpy_m1)/2;

== matlab function mechanization_ell_earth_noise/ellipsoide earth POS VEL mechanization2/make Cbn ==
  data: rpy input; Cbn output
function Cbn = make_Cbn(rpy)
%compute Cbn
Cz=[cos(rpy(3))     sin(rpy(3))     0; ...
    -sin(rpy(3))    cos(rpy(3))     0; ...
    0               0               1];

Cy=[cos(rpy(2))     0               -sin(rpy(2)); ...
    0               1               0; ...
    sin(rpy(2))     0               cos(rpy(2))];

Cx=[1               0               0;...
    0               cos(rpy(1))     sin(rpy(1)); ...
    0               -sin(rpy(1))    cos(rpy(1))];

Cbn = (Cx*Cy*Cz)';

== matlab function mechanization_ell_earth_noise/ellipsoide earth POS VEL mechanization3/MATLAB Function ==
  data: vel_n input; lat_dot output; prev_lat input; prev_h input; lon_dot output; h_dot output
function [lat_dot, lon_dot, h_dot] = ellipsoid_mechanization(vel_n, prev_lat, prev_h)

vel_N = vel_n(1);
vel_E = vel_n(2);
vel_D = vel_n(3);

% Constants WGS-84

re = 6378137;
eps = 0.0818191908426;
eps2 = eps^2;

phi = prev_lat;
h = prev_h;

sin2phi = sin(phi)^2;
den = 1 - eps2 * sin2phi ; 

R_N = re / (sqrt(den));
R_M = R_N * (1 - eps2)/(den);

lat_dot = vel_N / (R_M + h);
lon_dot = vel_E / (R_N + h) / cos(phi) ;
h_dot = - vel_D;

end
